simulink model "VCU_SW_2020"  (R2020b)
settings: Solver=FixedStepDiscrete  StartTime=0.0  StopTime=inf  FixedStep=1e-2  RelTol=1e-3
PreLoadFcn:
  | RTWConfigurationCB('preloadfcn', bdroot);
InitFcn:
  | loadvar_ttc500
undefined symbols (not defined in the file): BrkPedalTypes, CabMovModeTypes, cFuseTempSensAcc_X, cFuseTempSensAcc_Y, cFuseTempSensVal_X, cFuseTempSensVal_Y, cTMSTempSensVal_X, cTMSTempSensVal_Y, cTransferCaseSpeedRatio, diag_state, DoorsPositionTypes, dP_filter_Y, DriverOccClassSystemTypes, ErrorValueTypes, fatal_error_callback, IO_ADC_NO_RANGE, LadderStatusTypes, pAnalogCabRotSensAcc, pAnalogCabRotSensMaxVolt, pAnalogCabRotSensMinVolt, pAnalogCabRotSensRange, pAnalogCabRotSensZeroVolt, pBrkActivePress, pCabTiltSensAcc, pCabTiltSensMaxCur, pCabTiltSensMinCur, pDistanceCorrection, pECANManual_BPNEnable, pECANManual_BPNEnabler_Flag, pFilterSensAccRes, pHDirMaxDiffFrq, pHDirSensHighLvl, pHDirSensLowLvl, pMainGearRatio, pMaxFilterSensRes, pMaxFirstPedalSensValue, pMaxFuseTempSensRes, pMaxPressLoss, pMaxPressSensCurrent, pMaxPressValue, pMaxPressValueHydMotAndPump, pMaxPressValueParkDrain, pMaxSecondPedalSensValue, pMaxTempSensVoltage, pMaxTempValue, pMaxTMSTempSensRes, pMinFilterSensRes, pMinFirstPedalSensValue, pMinFuseTempSensRes, pMinPressLoss, pMinPressSensCurrent, pMinPressValue, pMinSecondPedalSensValue, pMinTempSensVoltage, pMinTempValue, pMinTMSTempSensRes, pMotorRingTeethNum, pPedalSensAccuracyPct, pPedalSensAccuracyVolt, pPressLossTreshhold ... (+20)
libraries: TTlibrary x270, canmsglib x127, simulink x88
(part 4 of 17)

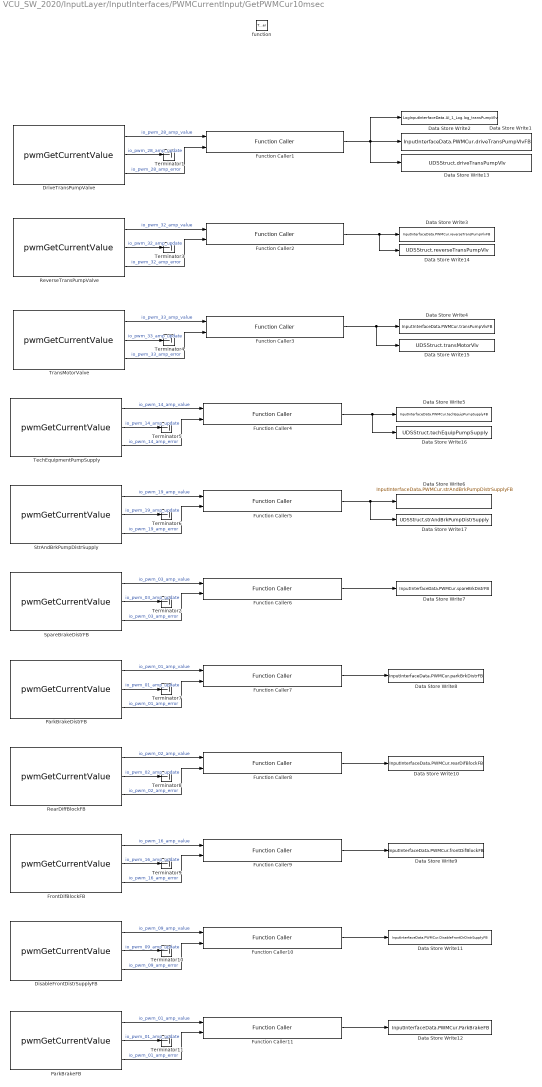
== system VCU_SW_2020/InputLayer/InputInterfaces/PWMCurrentInput/GetPWMCur10msec ==
  function : TriggerPort  TriggerType=function-call  VariantControl=Variant
  Data Store Write1 : DataStoreWrite  DataStoreName=InputInterfaceData  DataStoreElements=InputInterfaceData.PWMCur.driveTransPumpVlvFB
  Data Store Write10 : DataStoreWrite  DataStoreName=InputInterfaceData  DataStoreElements=InputInterfaceData.PWMCur.rearDifBlockFB
  Data Store Write11 : DataStoreWrite  DataStoreName=InputInterfaceData  DataStoreElements=InputInterfaceData.PWMCur.DisableFrontDrDistrSupplyFB
  Data Store Write12 : DataStoreWrite  DataStoreName=InputInterfaceData  DataStoreElements=InputInterfaceData.PWMCur.ParkBrakeFB
  Data Store Write13 : DataStoreWrite  DataStoreName=UDSStruct  DataStoreElements=UDSStruct.driveTransPumpVlv
  Data Store Write14 : DataStoreWrite  DataStoreName=UDSStruct  DataStoreElements=UDSStruct.reverseTransPumpVlv
  Data Store Write15 : DataStoreWrite  DataStoreName=UDSStruct  DataStoreElements=UDSStruct.transMotorVlv
  Data Store Write16 : DataStoreWrite  DataStoreName=UDSStruct  DataStoreElements=UDSStruct.techEquipPumpSupply
  Data Store Write17 : DataStoreWrite  DataStoreName=UDSStruct  DataStoreElements=UDSStruct.strAndBrkPumpDistrSupply
  Data Store Write2 : DataStoreWrite  DataStoreName=LogInputInterfaceData  DataStoreElements=LogInputInterfaceData.AI_1_Log.log_transPumpVlv
  Data Store Write3 : DataStoreWrite  DataStoreName=InputInterfaceData  DataStoreElements=InputInterfaceData.PWMCur.reverseTransPumpVlvFB
  Data Store Write4 : DataStoreWrite  DataStoreName=InputInterfaceData  DataStoreElements=InputInterfaceData.PWMCur.transPumpVlvFB
  Data Store Write5 : DataStoreWrite  DataStoreName=InputInterfaceData  DataStoreElements=InputInterfaceData.PWMCur.techEquipPumpSupplyFB
  Data Store Write6 : DataStoreWrite  DataStoreName=InputInterfaceData  DataStoreElements=InputInterfaceData.PWMCur.strAndBrkPumpDistrSupplyFB
  Data Store Write7 : DataStoreWrite  DataStoreName=InputInterfaceData  DataStoreElements=InputInterfaceData.PWMCur.spareBrkDistrFB
  Data Store Write8 : DataStoreWrite  DataStoreName=InputInterfaceData  DataStoreElements=InputInterfaceData.PWMCur.parkBrkDistrFB
  Data Store Write9 : DataStoreWrite  DataStoreName=InputInterfaceData  DataStoreElements=InputInterfaceData.PWMCur.frontDifBlockFB
  DisableFrontDistrSupplyFB : TTlibrary/PWM /pwmGetCurrentValue  pwm_channel=IO_PWM_09  io_error=on  sample_time=-1
      settings: SourceProductName=TT control 500 series
  DriveTransPumpValve : TTlibrary/PWM /pwmGetCurrentValue  pwm_channel=IO_PWM_28  io_error=on  sample_time=-1
      settings: SourceProductName=TT control 500 series
  FrontDifBlockFB : TTlibrary/PWM /pwmGetCurrentValue  pwm_channel=IO_PWM_16  io_error=on  sample_time=-1
      settings: SourceProductName=TT control 500 series
  Function Caller{1..11} (11 alike) : FunctionCaller  FunctionPrototype=finalValue = convPWMCurrData(rawValue,errorSts)  InputArgumentSpecifications=<Enter example>  OutputArgumentSpecifications=<Enter example>
  ParkBrakeDistrFB : TTlibrary/PWM /pwmGetCurrentValue  pwm_channel=IO_PWM_01  io_error=on  sample_time=-1
      settings: SourceProductName=TT control 500 series
  ParkBrakeFB : TTlibrary/PWM /pwmGetCurrentValue  pwm_channel=IO_PWM_01  io_error=on  sample_time=-1
      settings: SourceProductName=TT control 500 series
  RearDiffBlockFB : TTlibrary/PWM /pwmGetCurrentValue  pwm_channel=IO_PWM_02  io_error=on  sample_time=-1
      settings: SourceProductName=TT control 500 series
  ReverseTransPumpValve : TTlibrary/PWM /pwmGetCurrentValue  pwm_channel=IO_PWM_32  io_error=on  sample_time=-1
      settings: SourceProductName=TT control 500 series
  SpareBrakeDistrFB : TTlibrary/PWM /pwmGetCurrentValue  pwm_channel=IO_PWM_03  io_error=on  sample_time=-1
      settings: SourceProductName=TT control 500 series
  StrAndBrkPumpDistrSupply : TTlibrary/PWM /pwmGetCurrentValue  pwm_channel=IO_PWM_19  io_error=on  sample_time=-1
      settings: SourceProductName=TT control 500 series
  TechEquipmentPumpSupply : TTlibrary/PWM /pwmGetCurrentValue  pwm_channel=IO_PWM_14  io_error=on  sample_time=-1
      settings: SourceProductName=TT control 500 series
  Terminator{1..11} (11 alike) : Terminator
  TransMotorValve : TTlibrary/PWM /pwmGetCurrentValue  pwm_channel=IO_PWM_33  io_error=on  sample_time=-1
      settings: SourceProductName=TT control 500 series
  wires:
  Function Caller7/1 -> Data Store Write8/1
  ParkBrakeDistrFB/2 -> Terminator7/1  "io_pwm_01_amp_update"
  ParkBrakeDistrFB/1 -> Function Caller7/1  "io_pwm_01_amp_value"
  ParkBrakeDistrFB/3 -> Function Caller7/2  "io_pwm_01_amp_error"
  SpareBrakeDistrFB/3 -> Function Caller6/2  "io_pwm_03_amp_error"
  SpareBrakeDistrFB/1 -> Function Caller6/1  "io_pwm_03_amp_value"
  SpareBrakeDistrFB/2 -> Terminator2/1  "io_pwm_03_amp_update"
  Function Caller6/1 -> Data Store Write7/1
  Function Caller1/1 -> Data Store Write13/1, Data Store Write1/1, Data Store Write2/1
  StrAndBrkPumpDistrSupply/3 -> Function Caller5/2  "io_pwm_19_amp_error"
  Function Caller5/1 -> Data Store Write17/1, Data Store Write6/1
  StrAndBrkPumpDistrSupply/1 -> Function Caller5/1  "io_pwm_19_amp_value"
  StrAndBrkPumpDistrSupply/2 -> Terminator6/1  "io_pwm_19_amp_update"
  TechEquipmentPumpSupply/3 -> Function Caller4/2  "io_pwm_14_amp_error"
  Function Caller4/1 -> Data Store Write16/1, Data Store Write5/1
  TechEquipmentPumpSupply/1 -> Function Caller4/1  "io_pwm_14_amp_value"
  TechEquipmentPumpSupply/2 -> Terminator5/1  "io_pwm_14_amp_update"
  TransMotorValve/3 -> Function Caller3/2  "io_pwm_33_amp_error"
  Function Caller3/1 -> Data Store Write15/1, Data Store Write4/1
  TransMotorValve/1 -> Function Caller3/1  "io_pwm_33_amp_value"
  TransMotorValve/2 -> Terminator4/1  "io_pwm_33_amp_update"
  ReverseTransPumpValve/3 -> Function Caller2/2  "io_pwm_32_amp_error"
  Function Caller2/1 -> Data Store Write14/1, Data Store Write3/1
  ReverseTransPumpValve/1 -> Function Caller2/1  "io_pwm_32_amp_value"
  ReverseTransPumpValve/2 -> Terminator3/1  "io_pwm_32_amp_update"
  DriveTransPumpValve/3 -> Function Caller1/2  "io_pwm_28_amp_error"
  DriveTransPumpValve/1 -> Function Caller1/1  "io_pwm_28_amp_value"
  DriveTransPumpValve/2 -> Terminator1/1  "io_pwm_28_amp_update"
  RearDiffBlockFB/2 -> Terminator8/1  "io_pwm_02_amp_update"
  RearDiffBlockFB/3 -> Function Caller8/2  "io_pwm_02_amp_error"
  FrontDifBlockFB/3 -> Function Caller9/2  "io_pwm_16_amp_error"
  FrontDifBlockFB/1 -> Function Caller9/1  "io_pwm_16_amp_value"
  FrontDifBlockFB/2 -> Terminator9/1  "io_pwm_16_amp_update"
  RearDiffBlockFB/1 -> Function Caller8/1  "io_pwm_02_amp_value"
  Function Caller8/1 -> Data Store Write10/1
  Function Caller9/1 -> Data Store Write9/1
  Function Caller10/1 -> Data Store Write11/1
  DisableFrontDistrSupplyFB/2 -> Terminator10/1  "io_pwm_09_amp_update"
  DisableFrontDistrSupplyFB/1 -> Function Caller10/1  "io_pwm_09_amp_value"
  DisableFrontDistrSupplyFB/3 -> Function Caller10/2  "io_pwm_09_amp_error"
  ParkBrakeFB/3 -> Function Caller11/2  "io_pwm_01_amp_error"
  ParkBrakeFB/1 -> Function Caller11/1  "io_pwm_01_amp_value"
  ParkBrakeFB/2 -> Terminator11/1  "io_pwm_01_amp_update"
  Function Caller11/1 -> Data Store Write12/1

== system VCU_SW_2020/InputLayer/InputInterfaces/PWMCurrentInput/PWMCur10msecProc ==
  function : TriggerPort  TriggerType=function-call  VariantControl=Variant
  Constant12 : Constant  Value=pValveActiveCur
  Data Store Read : DataStoreRead  DataStoreName=InputInterfaceData  DataStoreElements=InputInterfaceData.PWMCur.DisableFrontDrDistrSupplyFB
  Data Store Read1 : DataStoreRead  DataStoreName=InputInterfaceData  DataStoreElements=InputInterfaceData.PWMCur.parkBrkDistrFB
  Data Store Read12 : DataStoreRead  DataStoreName=InputInterfaceData  DataStoreElements=InputInterfaceData.PWMCur.spareBrkDistrFB
  Data Store Read2 : DataStoreRead  DataStoreName=InputInterfaceData  DataStoreElements=InputInterfaceData.PWMCur.frontDifBlockFB
  Data Store Read3 : DataStoreRead  DataStoreName=InputInterfaceData  DataStoreElements=InputInterfaceData.PWMCur.rearDifBlockFB
  Data Store Write : DataStoreWrite  DataStoreName=InputFunctionsData  DataStoreElements=InputFunctionsData.frontDifBlockFB
  Data Store Write1 : DataStoreWrite  DataStoreName=InputFunctionsData  DataStoreElements=InputFunctionsData.spareBrkDistrFB
  Data Store Write2 : DataStoreWrite  DataStoreName=InputFunctionsData  DataStoreElements=InputFunctionsData.parkBrkDistrFB
  Data Store Write3 : DataStoreWrite  DataStoreName=InputFunctionsData  DataStoreElements=InputFunctionsData.rearDifBlockFB
  Data Store Write4 : DataStoreWrite  DataStoreName=InputFunctionsData  DataStoreElements=InputFunctionsData.DisableFrontDrDistrSupplyFB
  Data Store Write5 : DataStoreWrite  DataStoreName=InputFunctionsData  DataStoreElements=InputFunctionsData.parkBrakeFB
  Function Caller{,1..4} (5 alike) : FunctionCaller  FunctionPrototype=stt = ValveCurFBproc(pValveActiveCur,curFB)  InputArgumentSpecifications=<Enter example>  OutputArgumentSpecifications=<Enter example>
  MATLAB Function2 : MATLAB Function  TreatAsAtomicUnit=on
  Simulink Function : Subsystem  TreatAsAtomicUnit=on
  wires:
  Constant12/1 -> Function Caller1/1, Function Caller/1, Function Caller2/1, Function Caller3/1, Function Caller4/1
  Function Caller4/1 -> Data Store Write4/1
  Data Store Read/1 -> Function Caller4/2
  Data Store Read3/1 -> Function Caller3/2
  Data Store Read2/1 -> Function Caller2/2
  Function Caller3/1 -> Data Store Write3/1
  Function Caller2/1 -> Data Store Write/1
  Function Caller1/1 -> Data Store Write1/1
  Data Store Read1/1 -> Function Caller/2
  Function Caller/1 -> MATLAB Function2/1(sttRaw), Data Store Write2/1
  Data Store Read12/1 -> Function Caller1/2
  MATLAB Function2/1(sttInv) -> Data Store Write5/1

== system VCU_SW_2020/InputLayer/InputNetwork/InputCCAN/CCAN100msecProc1 ==
  function : TriggerPort  TriggerType=function-call  VariantControl=Variant
  CabMov buttons processing : Subsystem  TreatAsAtomicUnit=on
  InputTransSelect : Subsystem  TreatAsAtomicUnit=on
  JoystickRot : Subsystem  TreatAsAtomicUnit=on

== system VCU_SW_2020/InputLayer/InputNetwork/InputCCAN/CCAN10msecProc  ==
  function : TriggerPort  TriggerType=function-call  VariantControl=Variant

== system VCU_SW_2020/InputLayer/InputNetwork/InputCCAN/GetCCAN1000msec ==
  function : TriggerPort  TriggerType=function-call  VariantControl=Variant
  DD : Subsystem
  "Fuel Heater Data " : Subsystem
  LCMD : Subsystem
  LD : Subsystem
  OCSI : Subsystem
  VF : Subsystem

== system VCU_SW_2020/InputLayer/InputNetwork/InputCCAN/GetCCAN100msec ==
  note: КОСТЫЛЬ
  note: Вот тут тоже с типом данных матлаб функци брехня, посмотреть везде
  function : TriggerPort  TriggerType=function-call  VariantControl=Variant
  AUX_VLV_EST_CABIN : Subsystem
  BJM1 : Subsystem
  BJM2 : Subsystem
  CM1 : Subsystem
  CM3 : Subsystem
  CabinAuxiliaryStatus : Subsystem
  DC1 : Subsystem
  "Fan Rotation Direction Control " : Subsystem
  "Fan Rotation Direction Status " : Subsystem
  FuelTankAndFrameLock : Subsystem
  "Instrument Cluster Status " : Subsystem
  Left Big Pan Cmd : Subsystem
  Left Small Pan Cmd : Subsystem
  "OWW Status " : Subsystem
  PTO : Subsystem
  "Remote Brake Command " : Subsystem
  Right Small Pan Cmd : Subsystem
  TC1 : Subsystem

== system VCU_SW_2020/InputLayer/InputNetwork/InputCCAN/GetCCAN10msec ==
  function : TriggerPort  TriggerType=function-call  VariantControl=Variant
  CAN_Unpack_PLC_StateM : canmsglib/CAN Unpack  Commented=on  MsgList=(none)  MsgName=PLC_StateM  MsgIDType=Extended (29-bit identifier)  MsgIdentifier=419388800  MsgLength=5  SignalInfo={ 'PLC_V2G_StateM_SM9MesState', '16', '8', 'LE', 'unsigned', 'Standard', '0', '1', '0', '0', '255'; 'PLC_V2G_StateM_SM9Status', '24', '8', 'LE', 'unsigned', 'Standard', '0', '1', '0', '0', '255' }  IDPort=off  TimestampPort=off  ErrorPort=off  RemotePort=off  LengthPort=off  StatusPort=off  ApplyMinMax=off
  DataStoreWrite_PLC_StateM : DataStoreWrite  Commented=on  DataStoreName=InputNetworkData  DataStoreElements=InputNetworkData.ECAN.PLC.PLC_V2G_StateM_SM9MesState#InputNetworkData.ECAN.PLC.PLC_V2G_StateM_SM9Status
  Terminator : Terminator  Commented=on
  read_message_PLC_StateM : TTlibrary/CAN/read_message_name  Commented=on  channel=IO_CAN_CHANNEL_1  id_format=IO_CAN_EXT_FRAME  get_msg_info=off  message_names=there is no CAN Unpack blocks  message_info=|  id=419388800  ac_mask=536870911  retranslation=off  io_error=on  sample_time=-1
      | Message Name: PLC_StateM
      |  Message ID Type: Extended (29-bit identifier)
      |  Message ID: 419388800
      settings: SourceProductName=TT control 500 series
  wires:
  read_message_PLC_StateM/1 -> CAN_Unpack_PLC_StateM/1  "msg_419388800"
  read_message_PLC_StateM/2 -> Terminator/1  "handler_err_419388800"
  CAN_Unpack_PLC_StateM/1 -> DataStoreWrite_PLC_StateM/1
  CAN_Unpack_PLC_StateM/2 -> DataStoreWrite_PLC_StateM/2

== system VCU_SW_2020/InputLayer/InputNetwork/InputCCAN/GetCCAN200msec ==
  function : TriggerPort  TriggerType=function-call  VariantControl=Variant
  OWW : Subsystem

== system VCU_SW_2020/InputLayer/InputNetwork/InputCCAN/GetCCAN500msec ==
  function : TriggerPort  TriggerType=function-call  VariantControl=Variant
  EAC1 : Subsystem

== system VCU_SW_2020/InputLayer/InputNetwork/InputDiagCAN/GetDiagCAN10msec ==
  function : TriggerPort  TriggerType=function-call  VariantControl=Variant
  Data Store Write : DataStoreWrite  DataStoreName=UDSStruct  DataStoreElements=UDSStruct.readUDSmsgFlag
  MATLAB Function : MATLAB Function  TreatAsAtomicUnit=on
  Simulink Function : Subsystem  TreatAsAtomicUnit=on
  Simulink Function1 : Subsystem  TreatAsAtomicUnit=on
  Simulink Function2 : Subsystem  TreatAsAtomicUnit=on
  wires:
  MATLAB Function/1(ReadUDSmsgFlag) -> Data Store Write/1

== system VCU_SW_2020/InputLayer/InputNetwork/InputDiagCAN/GetDiagCAN10msec1 ==
  function : TriggerPort  TriggerType=function-call  VariantControl=Variant
  MATLAB Function : MATLAB Function  TreatAsAtomicUnit=on
  Simulink Function1 : Subsystem  TreatAsAtomicUnit=on
  Simulink Function2 : Subsystem  TreatAsAtomicUnit=on

== system VCU_SW_2020/InputLayer/InputNetwork/InputEngCAN/GetEngCAN1000msec ==
  function : TriggerPort  TriggerType=function-call  VariantControl=Variant
  CANUnpack_ECU_DLCC1 : canmsglib/CAN Unpack  MsgList=(none)  MsgName=ECU_DLCC1  MsgIDType=Extended (29-bit identifier)  MsgIdentifier=419235584  MsgLength=8  SignalInfo={ 'ECU_DLCC1_EngAirFiltRestrLampCmd', '22', '2', 'LE', 'unsigned', 'Standard', '0', '1', '0', '0', '3'; 'ECU_DLCC1_EngAmberWarnLampCmd', '2', '2', 'LE', 'unsigned', 'Standard', '0', '1', '0', '0', '3'; 'ECU_DLCC1_EngCoolLevLowLampCmd', '16', '2', 'LE', 'unsigned', 'Standard', '0', '1', '0', '0', '3'; 'ECU_DLCC1_EngCoolTempHiLampCmd', '14', '2', 'LE', 'unsigned', 'Standard', '0', '1', '0', '0', '3'; 'ECU_DLCC1_EngOilPressLowLampCmd', '12', '2', 'LE', 'unsigned', 'Standard', '0', '1', '0', '0', '3'; 'ECU_DLCC1_EngProtLampCmd', '0', '2', 'LE', 'unsigned', 'Standard', '0', '1', '0', '0', '3'; 'ECU_DLCC1_EngRedStopLampCmd', '4', '2', 'LE', 'unsigned', 'Standard', '0', '1', '0', '0', '3' }  IDPort=off  TimestampPort=off  ErrorPort=off  RemotePort=off  LengthPort=off  StatusPort=off  ApplyMinMax=off
  CANUnpack_ECU_ET1 : canmsglib/CAN Unpack  MsgList=(none)  MsgName=ECU_ET1  MsgIDType=Extended (29-bit identifier)  MsgIdentifier=419360256  MsgLength=8  SignalInfo={ 'ECU_ET1_EngCoolTemp', '0', '8', 'LE', 'unsigned', 'Standard', '0', '1', '-40', '-40', '210'; 'ECU_ET1_EngFuelTemp1', '8', '8', 'LE', 'unsigned', 'Standard', '0', '1', '-40', '-40', '210'; 'ECU_ET1_EngIntThOp', '56', '8', 'LE', 'unsigned', 'Standard', '0', '0.4', '0', '0', '100'; 'ECU_ET1_EngInterTemp', '48', '8', 'LE', 'unsigned', 'Standard', '0', '1', '-40', '-40', '210'; 'ECU_ET1_EngOilTemp1', '16', '16', 'LE', 'unsigned', 'Standard', '0', '0.03125', '-273', '-273', '1734.9688'; 'ECU_ET1_EngTurbOilTemp', '32', '16', 'LE', 'unsigned', 'Standard', '0', '0.03125', '-273', '-273', '1734.9688' }  IDPort=off  TimestampPort=off  ErrorPort=off  RemotePort=off  LengthPort=off  StatusPort=off  ApplyMinMax=off
  CANUnpack_ECU_ET2 : canmsglib/CAN Unpack  MsgList=(none)  MsgName=ECU_ET2  MsgIDType=Extended (29-bit identifier)  MsgIdentifier=419341312  MsgLength=8  SignalInfo={ 'ECU_ET2_EngECUTemp', '16', '16', 'LE', 'unsigned', 'Standard', '0', '0.03125', '-273', '-273', '1734.9688'; 'ECU_ET2_EngExGasRec1T', '48', '16', 'LE', 'unsigned', 'Standard', '0', '0.03125', '-273', '-273', '1734.9688'; 'ECU_ET2_EngExhGasRec1DP', '32', '16', 'LE', 'unsigned', 'Standard', '0', '0.0078125', '-250', '-250', '251.99'; 'ECU_ET2_EngOilTemp2', '0', '16', 'LE', 'unsigned', 'Standard', '0', '0.03125', '-273', '-273', '1734.9688' }  IDPort=off  TimestampPort=off  ErrorPort=off  RemotePort=off  LengthPort=off  StatusPort=off  ApplyMinMax=off
  CANUnpack_ECU_ET3 : canmsglib/CAN Unpack  MsgList=(none)  MsgName=ECU_THO  MsgIDType=Extended (29-bit identifier)  MsgIdentifier=419357952  MsgLength=8  SignalInfo={ 'EngTotalHours', '0', '32', 'LE', 'signed', 'Standard', '0', '0.05', '0', '0', '210554060.75' }  IDPort=off  TimestampPort=off  ErrorPort=off  RemotePort=off  LengthPort=off  StatusPort=off  ApplyMinMax=off
  CANUnpack_ECU_SHUTDN : canmsglib/CAN Unpack  MsgList=(none)  MsgName=ECU_SHUTDN  MsgIDType=Extended (29-bit identifier)  MsgIdentifier=419357696  MsgLength=8  SignalInfo={ 'ECU_SHUTDN_ACHighPrFanSw', '16', '2', 'LE', 'unsigned', 'Standard', '0', '1', '0', '0', '3'; 'ECU_SHUTDN_CoolLvlEngPrShSt', '60', '2', 'LE', 'unsigned', 'Standard', '0', '1', '0', '0', '3'; 'ECU_SHUTDN_EnIdShDAM', '2', '2', 'LE', 'unsigned', 'Standard', '0', '1', '0', '0', '3'; 'ECU_SHUTDN_EnIdShSE', '0', '2', 'LE', 'unsigned', 'Standard', '0', '1', '0', '0', '3'; 'ECU_SHUTDN_EnIdShTF', '14', '2', 'LE', 'unsigned', 'Standard', '0', '1', '0', '0', '3'; 'ECU_SHUTDN_EnIdShTO', '4', '2', 'LE', 'unsigned', 'Standard', '0', '1', '0', '0', '3'; 'ECU_SHUTDN_EnIdShTS', '6', '2', 'LE', 'unsigned', 'Standard', '0', '1', '0', '0', '3'; 'ECU_SHUTDN_EngAirShComSt', '52', '2', 'LE', 'unsigned', 'Standard', '0', '1', '0', '0', '3'; 'ECU_SHUTDN_EngAirShSt', '56', '2', 'LE', 'unsigned', 'Standard', '0', '1', '0', '0', '3'; 'ECU_SHUTDN_EngAlAckn', '48', '2', 'LE', 'unsigned', 'Standard', '0', '1', '0', '0', '3'; 'ECU_SHUTDN_EngAlOutComSt', '50', '2', 'LE', 'unsigned', 'Standard', '0', '1', '0', '0', '3'; 'ECU_SHUTDN_EngOverspTest', '54', '2', 'LE', 'unsigned', 'Standard', '0', '1', '0', '0', '3'; 'ECU_SHUTDN_EngProtSysAppSh', '34', '2', 'LE', 'unsigned', 'Standard', '0', '1', '0', '0', '3'; 'ECU_SHUTDN_EngProtSysConf', '46', '2', 'LE', 'unsigned', 'Standard', '0', '1', '0', '0', '3'; 'ECU_SHUTDN_EngProtSysShEng', '32', '2', 'LE', 'unsigned', 'Standard', '0', '1', '0', '0', '3'; 'ECU_SHUTDN_EngProtSysTimOver', '36', '2', 'LE', 'unsigned', 'Standard', '0', '1', '0', '0', '3'; 'ECU_SHUTDN_EngProtSysTimSt', '38', '2', 'LE', 'unsigned', 'Standard', '0', '1', '0', '0', '3'; 'ECU_SHUTDN_EngWaitStLam', '24', '2', 'LE', 'unsigned', 'Standard', '0', '1', '0', '0', '3'; 'ECU_SHUTDN_PTOShSE', '58', '2', 'LE', 'unsigned', 'Standard', '0', '1', '0', '0', '3'; 'ECU_SHUTDN_RefrHiPrSw', '20', '2', 'LE', 'unsigned', 'Standard', '0', '1', '0', '0', '3'; 'ECU_SHUTDN_RefrLowPrSw', '18', '2', 'LE', 'unsigned', 'Standard', '0', '1', '0', '0', '3' }  IDPort=off  TimestampPort=off  ErrorPort=off  RemotePort=off  LengthPort=off  StatusPort=off  ApplyMinMax=off
  CANUnpack_ECU_VEP1 : canmsglib/CAN Unpack  MsgList=(none)  MsgName=ECU_VEP1  MsgIDType=Extended (29-bit identifier)  MsgIdentifier=419362560  MsgLength=8  SignalInfo={ 'ECU_VEP1_AltCur', '8', '8', 'LE', 'unsigned', 'Standard', '0', '1', '-125', '-125', '125'; 'ECU_VEP1_BatPot', '32', '16', 'LE', 'unsigned', 'Standard', '0', '0.05', '0', '0', '3212.75'; 'ECU_VEP1_ChrgSysPot', '16', '16', 'LE', 'unsigned', 'Standard', '0', '0.05', '0', '0', '3212.75'; 'ECU_VEP1_KeyswPot', '48', '16', 'LE', 'unsigned', 'Standard', '0', '0.05', '0', '0', '3212.75'; 'ECU_VEP1_NetBatCur', '0', '8', 'LE', 'unsigned', 'Standard', '0', '1', '-125', '-125', '125' }  IDPort=off  TimestampPort=off  ErrorPort=off  RemotePort=off  LengthPort=off  StatusPort=off  ApplyMinMax=off
  Data Store Write : DataStoreWrite  DataStoreName=InputNetworkData  DataStoreElements=InputNetworkData.EngCAN.EngTotalHours
  Data Store Write1 : DataStoreWrite  DataStoreName=InputNetworkData  DataStoreElements=InputNetworkData.EngCAN.EngAirFiltRestrLampCmd#InputNetworkData.EngCAN.EngAmberWarnLampCmd#InputNetworkData.EngCAN.EngCoolLevLowLampCmd#InputNetworkData.EngCAN.EngCoolTempHiLampCmd#InputNetworkData.EngCAN.EngOilPressLowLampCmd#InputNetworkData.EngCAN.EngProtLampCmd#InputNetworkData.EngCAN.EngRedStopLampCmd
  Data Store Write2 : DataStoreWrite  Commented=on  DataStoreName=InputNetworkData  DataStoreElements=InputNetworkData.EngCAN.EngTotalHours
  Data Store Write4 : DataStoreWrite  DataStoreName=InputNetworkData  DataStoreElements=InputNetworkData.EngCAN.EngCoolTemp#InputNetworkData.EngCAN.EngFuelTemp1#InputNetworkData.EngCAN.EngIntThOp#InputNetworkData.EngCAN.EngInterTemp#InputNetworkData.EngCAN.EngOilTemp1#InputNetworkData.EngCAN.EngTurbOilTemp
  Data Store Write5 : DataStoreWrite  DataStoreName=InputNetworkData  DataStoreElements=InputNetworkData.EngCAN.EngECUTemp#InputNetworkData.EngCAN.EngExGasRec1T#InputNetworkData.EngCAN.EngExhGasRec1DP#InputNetworkData.EngCAN.EngOilTemp2
  Data Store Write6 : DataStoreWrite  DataStoreName=InputNetworkData  DataStoreElements=InputNetworkData.EngCAN.ACHighPrFanSw#InputNetworkData.EngCAN.CoolLvlEngPrShSt#InputNetworkData.EngCAN.EnIdShDAM#InputNetworkData.EngCAN.EnIdShSE#InputNetworkData.EngCAN.EnIdShTF#InputNetworkData.EngCAN.EnIdShTO#InputNetworkData.EngCAN.EnIdShTS#InputNetworkData.EngCAN.EngAirShComSt#InputNetworkData.EngCAN.EngAirShSt#InputNetworkData.EngCAN.EngAlAckn#InputNetworkData.EngCAN.EngAlOutComSt#InputNetworkData.EngCAN.EngOverspTest#InputNetworkData.EngCAN.EngProtSysAppSh#InputNetworkData.EngCAN.EngProtSysConf#InputNetworkData.EngCAN.EngProtSysShEng#InputNetworkData.EngCAN.EngProtSysTimOver#InputNetworkData.EngCAN.EngProtSysTimSt#InputNetworkData.EngCAN.EngWaitStLam#InputNetworkData.EngCAN.PTOShSE#InputNetworkData.EngCAN.RefrHiPrSw#InputNetworkData.EngCAN.RefrLowPrSw
  Data Store Write7 : DataStoreWrite  DataStoreName=InputNetworkData  DataStoreElements=InputNetworkData.EngCAN.AltCur#InputNetworkData.EngCAN.BatPot#InputNetworkData.EngCAN.ChrgSysPot#InputNetworkData.EngCAN.KeyswPot#InputNetworkData.EngCAN.NetBatCur
  Function Caller1 : FunctionCaller  FunctionPrototype=rawValue = convUintPinToenumStt(uintValue)  InputArgumentSpecifications=<Enter example>  OutputArgumentSpecifications=<Enter example>
  MATLAB Function : MATLAB Function  TreatAsAtomicUnit=on
  Terminator{,1..5} (6 alike) : Terminator
  read_DLCC1 : TTlibrary/CAN/read_message_name  channel=IO_CAN_CHANNEL_2  id_format=IO_CAN_EXT_FRAME  get_msg_info=off  message_names=there is no CAN Unpack blocks  message_info=|  id=419235584  ac_mask=536870911  retranslation=off  io_error=on  sample_time=-1
      | Message Name: ECU_VEP1
      |  Message ID Type: Extended (29-bit identifier)
      |  Message ID: 419362560
      settings: SourceProductName=TT control 500 series
  read_DLCC2 : TTlibrary/CAN/read_message_name  channel=IO_CAN_CHANNEL_2  id_format=IO_CAN_EXT_FRAME  get_msg_info=off  message_names=there is no CAN Unpack blocks  message_info=|  id=419357952  ac_mask=536870911  retranslation=off  io_error=on  sample_time=-1
      | Message Name: ECU_VEP1
      |  Message ID Type: Extended (29-bit identifier)
      |  Message ID: 419362560
      settings: SourceProductName=TT control 500 series
  read_ECU_ET1 : TTlibrary/CAN/read_message_name  channel=IO_CAN_CHANNEL_2  id_format=IO_CAN_EXT_FRAME  get_msg_info=off  message_names=there is no CAN Unpack blocks  message_info=|  id=419360256  ac_mask=536870911  retranslation=off  io_error=on  sample_time=-1
      | Message Name: ECU_ET1
      |  Message ID Type: Extended (29-bit identifier)
      |  Message ID: 419360256
      settings: SourceProductName=TT control 500 series
  read_ECU_ET2 : TTlibrary/CAN/read_message_name  channel=IO_CAN_CHANNEL_2  id_format=IO_CAN_EXT_FRAME  get_msg_info=off  message_names=there is no CAN Unpack blocks  message_info=|  id=419341312  ac_mask=536870911  retranslation=off  io_error=on  sample_time=-1
      | Message Name: ECU_ET2
      |  Message ID Type: Extended (29-bit identifier)
      |  Message ID: 419341312
      settings: SourceProductName=TT control 500 series
  read_ECU_SHUTDN : TTlibrary/CAN/read_message_name  channel=IO_CAN_CHANNEL_2  id_format=IO_CAN_EXT_FRAME  get_msg_info=off  message_names=there is no CAN Unpack blocks  message_info=|  id=419357696  ac_mask=536870911  retranslation=off  io_error=on  sample_time=-1
      | Message Name: ECU_SHUTDN
      |  Message ID Type: Extended (29-bit identifier)
      |  Message ID: 419357696
      settings: SourceProductName=TT control 500 series
  read_ECU_VEP1 : TTlibrary/CAN/read_message_name  channel=IO_CAN_CHANNEL_2  id_format=IO_CAN_EXT_FRAME  get_msg_info=off  message_names=there is no CAN Unpack blocks  message_info=|  id=419362560  ac_mask=536870911  retranslation=off  io_error=on  sample_time=-1
      | Message Name: ECU_VEP1
      |  Message ID Type: Extended (29-bit identifier)
      |  Message ID: 419362560
      settings: SourceProductName=TT control 500 series
  wires:
  CANUnpack_ECU_ET3/1 -> Data Store Write/1
  read_DLCC2/2 -> Terminator5/1  "handler_err_419357952"
  read_DLCC2/1 -> CANUnpack_ECU_ET3/1  "msg_419357952"
  CANUnpack_ECU_DLCC1/7 -> Data Store Write1/7
  CANUnpack_ECU_DLCC1/6 -> Data Store Write1/6
  CANUnpack_ECU_DLCC1/5 -> Data Store Write1/5
  CANUnpack_ECU_DLCC1/4 -> Data Store Write1/4
  CANUnpack_ECU_DLCC1/3 -> Data Store Write1/3
  CANUnpack_ECU_DLCC1/2 -> Data Store Write1/2
  CANUnpack_ECU_DLCC1/1 -> Data Store Write1/1
  read_DLCC1/1 -> CANUnpack_ECU_DLCC1/1  "msg_419235584"
  read_DLCC1/2 -> Terminator4/1  "handler_err_419235584"
  MATLAB Function/1(coolLvlState) -> Data Store Write6/2
  CANUnpack_ECU_ET1/5 -> Data Store Write4/5
  Function Caller1/1 -> Data Store Write6/18
  read_ECU_VEP1/2 -> Terminator3/1  "handler_err_419362560"
  read_ECU_SHUTDN/2 -> Terminator2/1  "handler_err_419357696"
  read_ECU_ET2/2 -> Terminator1/1  "handler_err_419341312"
  read_ECU_ET1/2 -> Terminator/1  "handler_err_419360256"
  CANUnpack_ECU_SHUTDN/13 -> Data Store Write6/13
  CANUnpack_ECU_ET1/3 -> Data Store Write4/3
  CANUnpack_ECU_ET2/1 -> Data Store Write5/1
  CANUnpack_ECU_VEP1/2 -> Data Store Write7/2
  CANUnpack_ECU_SHUTDN/1 -> Data Store Write6/1
  CANUnpack_ECU_VEP1/1 -> Data Store Write7/1
  CANUnpack_ECU_ET1/4 -> Data Store Write4/4
  CANUnpack_ECU_SHUTDN/3 -> Data Store Write6/3
  CANUnpack_ECU_VEP1/5 -> Data Store Write7/5
  CANUnpack_ECU_SHUTDN/2 -> MATLAB Function/1(Value)
  CANUnpack_ECU_ET2/2 -> Data Store Write5/2
  CANUnpack_ECU_ET1/2 -> Data Store Write4/2
  CANUnpack_ECU_ET2/3 -> Data Store Write5/3
  CANUnpack_ECU_ET2/4 -> Data Store Write5/4
  CANUnpack_ECU_SHUTDN/5 -> Data Store Write6/5
  CANUnpack_ECU_SHUTDN/6 -> Data Store Write6/6
  CANUnpack_ECU_SHUTDN/8 -> Data Store Write6/8
  CANUnpack_ECU_SHUTDN/16 -> Data Store Write6/16
  CANUnpack_ECU_SHUTDN/9 -> Data Store Write6/9
  CANUnpack_ECU_SHUTDN/11 -> Data Store Write6/11
  CANUnpack_ECU_SHUTDN/10 -> Data Store Write6/10
  CANUnpack_ECU_SHUTDN/14 -> Data Store Write6/14
  CANUnpack_ECU_ET1/6 -> Data Store Write4/6
  CANUnpack_ECU_SHUTDN/15 -> Data Store Write6/15
  CANUnpack_ECU_SHUTDN/18 -> Function Caller1/1
  CANUnpack_ECU_SHUTDN/21 -> Data Store Write6/21
  CANUnpack_ECU_VEP1/3 -> Data Store Write7/3
  CANUnpack_ECU_VEP1/4 -> Data Store Write7/4
  CANUnpack_ECU_ET1/1 -> Data Store Write4/1
  CANUnpack_ECU_SHUTDN/12 -> Data Store Write6/12
  CANUnpack_ECU_SHUTDN/17 -> Data Store Write6/17
  CANUnpack_ECU_SHUTDN/20 -> Data Store Write6/20
  read_ECU_ET1/1 -> CANUnpack_ECU_ET1/1  "msg_419360256"
  read_ECU_SHUTDN/1 -> CANUnpack_ECU_SHUTDN/1  "msg_419357696"
  CANUnpack_ECU_SHUTDN/19 -> Data Store Write6/19
  CANUnpack_ECU_SHUTDN/4 -> Data Store Write6/4
  read_ECU_VEP1/1 -> CANUnpack_ECU_VEP1/1  "msg_419362560"
  CANUnpack_ECU_SHUTDN/7 -> Data Store Write6/7
  read_ECU_ET2/1 -> CANUnpack_ECU_ET2/1  "msg_419341312"

== system VCU_SW_2020/InputLayer/InputNetwork/InputEngCAN/GetEngCAN100msec ==
  function : TriggerPort  TriggerType=function-call  VariantControl=Variant
  CANUnpack_ECU_EEC1 : canmsglib/CAN Unpack  MsgList=(none)  MsgName=ECU_EEC1  MsgIDType=Extended (29-bit identifier)  MsgIdentifier=217056256  MsgLength=8  SignalInfo={ 'ECU_EEC1_ActEngPTrq', '16', '8', 'LE', 'unsigned', 'Standard', '0', '1', '-125', '-125', '125'; 'ECU_EEC1_ActEngPTrqHighRes', '4', '4', 'LE', 'unsigned', 'Standard', '0', '0.125', '0', '0', '0.875'; 'ECU_EEC1_DrDemEngPTrq', '8', '8', 'LE', 'unsigned', 'Standard', '0', '1', '-125', '-125', '125'; 'ECU_EEC1_EnStrtM', '48', '4', 'LE', 'unsigned', 'Standard', '0', '1', '0', '0', '15'; 'ECU_EEC1_EngDemPercTrq', '56', '8', 'LE', 'unsigned', 'Standard', '0', '1', '-125', '-125', '125'; 'ECU_EEC1_EngSpd', '24', '16', 'LE', 'unsigned', 'Standard', '0', '0.125', '0', '0', '8031.875'; 'ECU_EEC1_EngTrqM', '0', '4', 'LE', 'unsigned', 'Standard', '0', '1', '0', '0', '15'; 'ECU_EEC1_SrsAdr', '40', '8', 'LE', 'unsigned', 'Standard', '0', '1', '0', '0', '255' }  IDPort=off  TimestampPort=off  ErrorPort=off  RemotePort=off  LengthPort=off  StatusPort=off  ApplyMinMax=off
  CANUnpack_ECU_LFE1 : canmsglib/CAN Unpack  MsgList=(none)  MsgName=ECU_LFE1  MsgIDType=Extended (29-bit identifier)  MsgIdentifier=419361280  MsgLength=8  SignalInfo={ 'ECU_LFE1_EngAvrFE', '32', '16', 'LE', 'unsigned', 'Standard', '0', '0.0019531', '0', '0', '125.5'; 'ECU_LFE1_EngFuelRate', '0', '16', 'LE', 'unsigned', 'Standard', '0', '0.05', '0', '0', '3212.75'; 'ECU_LFE1_EngInstFE', '16', '16', 'LE', 'unsigned', 'Standard', '0', '0.0019531', '0', '0', '125.5'; 'ECU_LFE1_EngThrVlv1Pos', '48', '8', 'LE', 'unsigned', 'Standard', '0', '0.4', '0', '0', '100'; 'ECU_LFE1_EngThrVlv2Pos', '56', '8', 'LE', 'unsigned', 'Standard', '0', '0.4', '0', '0', '100' }  IDPort=off  TimestampPort=off  ErrorPort=off  RemotePort=off  LengthPort=off  StatusPort=off  ApplyMinMax=off
  CANUnpack_ECU_TPCM : canmsglib/CAN Unpack  Commented=on  MsgList=(none)  MsgName=ECU_TPCM  MsgIDType=Extended (29-bit identifier)  MsgIdentifier=418184960  MsgLength=8  SignalInfo={ 'ECU_TPCM_ContrByte', '0', '8', 'LE', 'unsigned', 'Standard', '0', '1', '0', '0', '255'; 'ECU_TPCM_MaxNumofPak', '32', '8', 'LE', 'unsigned', 'Standard', '0', '1', '0', '2', '255'; 'ECU_TPCM_NextPakNum', '48', '8', 'LE', 'unsigned', 'Standard', '0', '1', '0', '1', '255'; 'ECU_TPCM_NumPakCanSent', '40', '8', 'LE', 'unsigned', 'Standard', '0', '1', '0', '0', '255'; 'ECU_TPCM_SeqNum', '56', '8', 'LE', 'unsigned', 'Standard', '0', '1', '0', '1', '255'; 'ECU_TPCM_TotMesSize', '8', '16', 'LE', 'unsigned', 'Standard', '0', '1', '0', '9', '1785'; 'ECU_TPCM_TotNumofPak', '24', '8', 'LE', 'unsigned', 'Standard', '0', '1', '0', '2', '255' }  IDPort=off  TimestampPort=off  ErrorPort=off  RemotePort=off  LengthPort=off  StatusPort=off  ApplyMinMax=off
  CANUnpack_ECU_TPDT : canmsglib/CAN Unpack  Commented=on  MsgList=(none)  MsgName=ECU_TPDT  MsgIDType=Extended (29-bit identifier)  MsgIdentifier=418119424  MsgLength=8  SignalInfo={ 'ECU_TPDT_EMS_SeqNum', '0', '8', 'LE', 'unsigned', 'Standard', '0', '1', '0', '1', '255'; 'ECU_TPDT_EMS_byte1', '8', '8', 'LE', 'unsigned', 'Standard', '0', '1', '0', '0', '255'; 'ECU_TPDT_EMS_byte2', '16', '8', 'LE', 'unsigned', 'Standard', '0', '1', '0', '0', '255'; 'ECU_TPDT_EMS_byte3', '24', '8', 'LE', 'unsigned', 'Standard', '0', '1', '0', '0', '255'; 'ECU_TPDT_EMS_byte4', '32', '8', 'LE', 'unsigned', 'Standard', '0', '1', '0', '0', '255'; 'ECU_TPDT_EMS_byte5', '40', '8', 'LE', 'unsigned', 'Standard', '0', '1', '0', '0', '7.20575940379279e+16'; 'ECU_TPDT_EMS_byte6', '48', '8', 'LE', 'unsigned', 'Standard', '0', '1', '0', '0', '255'; 'ECU_TPDT_EMS_byte7', '56', '8', 'LE', 'unsigned', 'Standard', '0', '1', '0', '0', '255' }  IDPort=off  TimestampPort=off  ErrorPort=off  RemotePort=off  LengthPort=off  StatusPort=off  ApplyMinMax=off
  Data Store Write4 : DataStoreWrite  DataStoreName=InputNetworkData  DataStoreElements=InputNetworkData.EngCAN.ActEngPTrq#InputNetworkData.EngCAN.ActEngPTrqHighRes#InputNetworkData.EngCAN.DrDemEngPTrq#InputNetworkData.EngCAN.EnStrtM#InputNetworkData.EngCAN.EngDemPercTrq#InputNetworkData.EngCAN.EngSpd#InputNetworkData.EngCAN.EngTrqM#InputNetworkData.EngCAN.SrsAdr
  Data Store Write5 : DataStoreWrite  DataStoreName=InputNetworkData  DataStoreElements=InputNetworkData.EngCAN.EngAvrFE#InputNetworkData.EngCAN.EngFuelRate#InputNetworkData.EngCAN.EngInstFE#InputNetworkData.EngCAN.EngThrVlv1Pos#InputNetworkData.EngCAN.EngThrVlv2Pos
  Data Store Write6 : DataStoreWrite  Commented=on  DataStoreName=InputNetworkData  DataStoreElements=InputNetworkData.EngCAN.ContrByte#InputNetworkData.EngCAN.MaxNumofPak#InputNetworkData.EngCAN.NextPakNum#InputNetworkData.EngCAN.NumPakCanSent#InputNetworkData.EngCAN.SeqNum#InputNetworkData.EngCAN.TotMesSize#InputNetworkData.EngCAN.TotNumofPak
  Data Store Write7 : DataStoreWrite  Commented=on  DataStoreName=InputNetworkData  DataStoreElements=InputNetworkData.EngCAN.EMS_SeqNum#InputNetworkData.EngCAN.EMS_byte1#InputNetworkData.EngCAN.EMS_byte2#InputNetworkData.EngCAN.EMS_byte3#InputNetworkData.EngCAN.EMS_byte4#InputNetworkData.EngCAN.EMS_byte5#InputNetworkData.EngCAN.EMS_byte6#InputNetworkData.EngCAN.EMS_byte7
  Data Type Conversion : DataTypeConversion  OutDataTypeStr=int8
  Data Type Conversion1 : DataTypeConversion  OutDataTypeStr=int8
  Data Type Conversion2 : DataTypeConversion  OutDataTypeStr=int8
  Terminator : Terminator
  Terminator1 : Terminator
  Terminator2 : Terminator  Commented=on
  Terminator3 : Terminator  Commented=on
  calcEnStrtM : MATLAB Function  TreatAsAtomicUnit=on
  read_ECU_EEC1 : TTlibrary/CAN/read_message_name  channel=IO_CAN_CHANNEL_2  id_format=IO_CAN_EXT_FRAME  get_msg_info=off  message_names=there is no CAN Unpack blocks  message_info=|  id=217056256  ac_mask=536870911  retranslation=off  io_error=on  sample_time=-1
      | Message Name: ECU_EEC1
      |  Message ID Type: Extended (29-bit identifier)
      |  Message ID: 217056256
      settings: SourceProductName=TT control 500 series
  read_ECU_LFE1 : TTlibrary/CAN/read_message_name  channel=IO_CAN_CHANNEL_2  id_format=IO_CAN_EXT_FRAME  get_msg_info=off  message_names=there is no CAN Unpack blocks  message_info=|  id=419361280  ac_mask=536870911  retranslation=off  io_error=on  sample_time=-1
      | Message Name: ECU_LFE1
      |  Message ID Type: Extended (29-bit identifier)
      |  Message ID: 419361280
      settings: SourceProductName=TT control 500 series
  read_ECU_TPCM : TTlibrary/CAN/read_message_name  Commented=on  channel=IO_CAN_CHANNEL_2  id_format=IO_CAN_EXT_FRAME  get_msg_info=off  message_names=there is no CAN Unpack blocks  message_info=|  id=418184960  ac_mask=536870911  retranslation=off  io_error=on  sample_time=-1
      | Message Name: ECU_TPCM
      |  Message ID Type: Extended (29-bit identifier)
      |  Message ID: 418184960
      settings: SourceProductName=TT control 500 series
  read_ECU_TPDT : TTlibrary/CAN/read_message_name  Commented=on  channel=IO_CAN_CHANNEL_2  id_format=IO_CAN_EXT_FRAME  get_msg_info=off  message_names=there is no CAN Unpack blocks  message_info=|  id=418119424  ac_mask=536870911  retranslation=off  io_error=on  sample_time=-1
      | Message Name: ECU_TPDT
      |  Message ID Type: Extended (29-bit identifier)
      |  Message ID: 418119424
      settings: SourceProductName=TT control 500 series
  wires:
  CANUnpack_ECU_EEC1/6 -> Data Store Write4/6
  CANUnpack_ECU_EEC1/7 -> Data Store Write4/7
  calcEnStrtM/1(operatingMode) -> Data Store Write4/4
  read_ECU_TPDT/2 -> Terminator3/1  "handler_err_418119424"
  read_ECU_TPCM/2 -> Terminator2/1  "handler_err_418184960"
  read_ECU_LFE1/2 -> Terminator1/1  "handler_err_419361280"
  read_ECU_EEC1/2 -> Terminator/1  "handler_err_217056256"
  CANUnpack_ECU_EEC1/5 -> Data Type Conversion2/1
  CANUnpack_ECU_TPCM/1 -> Data Store Write6/1
  CANUnpack_ECU_EEC1/3 -> Data Type Conversion1/1
  CANUnpack_ECU_TPCM/5 -> Data Store Write6/5
  CANUnpack_ECU_TPDT/3 -> Data Store Write7/3
  CANUnpack_ECU_EEC1/2 -> Data Store Write4/2
  CANUnpack_ECU_TPDT/2 -> Data Store Write7/2
  CANUnpack_ECU_LFE1/2 -> Data Store Write5/2
  CANUnpack_ECU_TPDT/1 -> Data Store Write7/1
  CANUnpack_ECU_TPCM/3 -> Data Store Write6/3
  CANUnpack_ECU_EEC1/4 -> calcEnStrtM/1(Value)
  CANUnpack_ECU_TPDT/6 -> Data Store Write7/6
  CANUnpack_ECU_LFE1/4 -> Data Store Write5/4
  CANUnpack_ECU_TPCM/6 -> Data Store Write6/6
  CANUnpack_ECU_TPCM/2 -> Data Store Write6/2
  CANUnpack_ECU_EEC1/8 -> Data Store Write4/8
  CANUnpack_ECU_TPDT/8 -> Data Store Write7/8
  read_ECU_EEC1/1 -> CANUnpack_ECU_EEC1/1  "msg_217056256"
  CANUnpack_ECU_TPDT/4 -> Data Store Write7/4
  CANUnpack_ECU_TPDT/5 -> Data Store Write7/5
  CANUnpack_ECU_TPCM/4 -> Data Store Write6/4
  CANUnpack_ECU_LFE1/3 -> Data Store Write5/3
  read_ECU_TPCM/1 -> CANUnpack_ECU_TPCM/1  "msg_418184960"
  CANUnpack_ECU_TPDT/7 -> Data Store Write7/7
  CANUnpack_ECU_TPCM/7 -> Data Store Write6/7
  read_ECU_LFE1/1 -> CANUnpack_ECU_LFE1/1  "msg_419361280"
  CANUnpack_ECU_LFE1/5 -> Data Store Write5/5
  CANUnpack_ECU_EEC1/1 -> Data Type Conversion/1
  CANUnpack_ECU_LFE1/1 -> Data Store Write5/1
  read_ECU_TPDT/1 -> CANUnpack_ECU_TPDT/1  "msg_418119424"
  Data Type Conversion/1 -> Data Store Write4/1
  Data Type Conversion1/1 -> Data Store Write4/3
  Data Type Conversion2/1 -> Data Store Write4/5

== system VCU_SW_2020/InputLayer/InputNetwork/InputEngCAN/GetEngCAN250msec ==
  function : TriggerPort  TriggerType=function-call  VariantControl=Variant
  CANUnpack_ECU_EEC3 : canmsglib/CAN Unpack  MsgList=(none)  MsgName=ECU_EEC3  MsgIDType=Extended (29-bit identifier)  MsgIdentifier=419356416  MsgLength=8  SignalInfo={ 'ECU_EEC3_Aft1ExDP', '58', '2', 'LE', 'unsigned', 'Standard', '0', '1', '0', '0', '3'; 'ECU_EEC3_Aft1ExGasMasFl', '40', '16', 'LE', 'unsigned', 'Standard', '0', '0.2', '0', '0', '12851'; 'ECU_EEC3_Aft1IntDP', '56', '2', 'LE', 'unsigned', 'Standard', '0', '1', '0', '0', '3'; 'ECU_EEC3_Aft2ExDP', '62', '2', 'LE', 'unsigned', 'Standard', '0', '1', '0', '0', '3'; 'ECU_EEC3_Aft2IntDP', '60', '2', 'LE', 'unsigned', 'Standard', '0', '1', '0', '0', '3'; 'ECU_EEC3_EngDesOpSpd', '8', '16', 'LE', 'unsigned', 'Standard', '0', '0.125', '0', '0', '8031.875'; 'ECU_EEC3_EngDesOpSpdAA', '24', '8', 'LE', 'unsigned', 'Standard', '0', '1', '0', '0', '250'; 'ECU_EEC3_EstEngParLos', '32', '8', 'LE', 'unsigned', 'Standard', '0', '1', '-125', '-125', '125'; 'ECU_EEC3_NomFrPT', '0', '8', 'LE', 'unsigned', 'Standard', '0', '1', '-125', '-125', '125' }  IDPort=off  TimestampPort=off  ErrorPort=off  RemotePort=off  LengthPort=off  StatusPort=off  ApplyMinMax=off
  Data Store Write4 : DataStoreWrite  DataStoreName=InputNetworkData  DataStoreElements=InputNetworkData.EngCAN.Aft1ExDP#InputNetworkData.EngCAN.Aft1ExGasMasFl#InputNetworkData.EngCAN.Aft1IntDP#InputNetworkData.EngCAN.Aft2ExDP#InputNetworkData.EngCAN.Aft2IntDP#InputNetworkData.EngCAN.EngDesOpSpd#InputNetworkData.EngCAN.EngDesOpSpdAA#InputNetworkData.EngCAN.EstEngParLos#InputNetworkData.EngCAN.NomFrPT
  Terminator : Terminator
  read_ECU_EEC3 : TTlibrary/CAN/read_message_name  channel=IO_CAN_CHANNEL_2  id_format=IO_CAN_EXT_FRAME  get_msg_info=off  message_names=there is no CAN Unpack blocks  message_info=|  id=419356416  ac_mask=536870911  retranslation=off  io_error=on  sample_time=-1
      | Message Name: ECU_EEC3
      |  Message ID Type: Extended (29-bit identifier)
      |  Message ID: 419356416
      settings: SourceProductName=TT control 500 series
  wires:
  read_ECU_EEC3/2 -> Terminator/1  "handler_err_419356416"
  CANUnpack_ECU_EEC3/2 -> Data Store Write4/2
  read_ECU_EEC3/1 -> CANUnpack_ECU_EEC3/1  "msg_419356416"
  CANUnpack_ECU_EEC3/4 -> Data Store Write4/4
  CANUnpack_ECU_EEC3/7 -> Data Store Write4/7
  CANUnpack_ECU_EEC3/1 -> Data Store Write4/1
  CANUnpack_ECU_EEC3/6 -> Data Store Write4/6
  CANUnpack_ECU_EEC3/9 -> Data Store Write4/9
  CANUnpack_ECU_EEC3/8 -> Data Store Write4/8
  CANUnpack_ECU_EEC3/3 -> Data Store Write4/3
  CANUnpack_ECU_EEC3/5 -> Data Store Write4/5

== system VCU_SW_2020/InputLayer/InputNetwork/InputEngCAN/GetEngCAN500msec ==
  function : TriggerPort  TriggerType=function-call  VariantControl=Variant
  CANUnpack_ECU_EFL_P1 : canmsglib/CAN Unpack  MsgList=(none)  MsgName=ECU_EFL_P1  MsgIDType=Extended (29-bit identifier)  MsgIdentifier=419360512  MsgLength=8  SignalInfo={ 'EngCoolLevel', '56', '8', 'LE', 'unsigned', 'Standard', '0', '0.4', '0', '0', '100'; 'EngOilPress', '24', '8', 'LE', 'unsigned', 'Standard', '0', '4', '0', '0', '1000' }  IDPort=off  TimestampPort=off  ErrorPort=off  RemotePort=off  LengthPort=off  StatusPort=off  ApplyMinMax=off
  Data Store Write2 : DataStoreWrite  DataStoreName=InputNetworkData  DataStoreElements=InputNetworkData.EngCAN.EngCoolLevel#InputNetworkData.EngCAN.EngOilPress
  Terminator5 : Terminator
  read_ECU_EFL_P1 : TTlibrary/CAN/read_message_name  channel=IO_CAN_CHANNEL_2  id_format=IO_CAN_EXT_FRAME  get_msg_info=off  message_names=there is no CAN Unpack blocks  message_info=|  id=419360512  ac_mask=536870911  retranslation=off  io_error=on  sample_time=-1
      | Message Name: ECU_VEP1
      |  Message ID Type: Extended (29-bit identifier)
      |  Message ID: 419362560
      settings: SourceProductName=TT control 500 series
  wires:
  CANUnpack_ECU_EFL_P1/2 -> Data Store Write2/2
  CANUnpack_ECU_EFL_P1/1 -> Data Store Write2/1
  read_ECU_EFL_P1/2 -> Terminator5/1  "handler_err_419360512"
  read_ECU_EFL_P1/1 -> CANUnpack_ECU_EFL_P1/1  "msg_419360512"

== system VCU_SW_2020/InputLayer/InputNetwork/InputEngCAN/GetEngCAN50msec ==
  function : TriggerPort  TriggerType=function-call  VariantControl=Variant
  CANUnpack_ECU_EEC2 : canmsglib/CAN Unpack  MsgList=(none)  MsgName=ECU_EEC2  MsgIDType=Extended (29-bit identifier)  MsgIdentifier=217056000  MsgLength=8  SignalInfo={ 'ECU_EEC2_AccPed1LIS', '0', '2', 'LE', 'unsigned', 'Standard', '0', '1', '0', '0', '3'; 'ECU_EEC2_AccPed2LIS', '6', '2', 'LE', 'unsigned', 'Standard', '0', '1', '0', '0', '3'; 'ECU_EEC2_AccPedKS', '2', '2', 'LE', 'unsigned', 'Standard', '0', '1', '0', '0', '3'; 'ECU_EEC2_AccPedPos1', '8', '8', 'LE', 'unsigned', 'Standard', '0', '0.4', '0', '0', '100'; 'ECU_EEC2_AccPedPos2', '32', '8', 'LE', 'unsigned', 'Standard', '0', '0.4', '0', '0', '100'; 'ECU_EEC2_ActMacAvEngTrq', '48', '8', 'LE', 'unsigned', 'Standard', '0', '0.4', '0', '0', '100'; 'ECU_EEC2_DPF', '44', '2', 'LE', 'unsigned', 'Standard', '0', '1', '0', '0', '3'; 'ECU_EEC2_EngPercLoatCS', '16', '8', 'LE', 'unsigned', 'Standard', '0', '1', '0', '0', '250'; 'ECU_EEC2_EstPumpTrq', '56', '8', 'LE', 'unsigned', 'Standard', '0', '1', '-125', '-125', '125'; 'ECU_EEC2_MomEngMaxPwr', '42', '2', 'LE', 'unsigned', 'Standard', '0', '1', '0', '0', '3'; 'ECU_EEC2_RdSpdLS', '4', '2', 'LE', 'unsigned', 'Standard', '0', '1', '0', '0', '3'; 'ECU_EEC2_RemAccPedPos', '24', '8', 'LE', 'unsigned', 'Standard', '0', '0.4', '0', '0', '100'; 'ECU_EEC2_SCR', '46', '2', 'LE', 'unsigned', 'Standard', '0', '1', '0', '0', '3'; 'ECU_EEC2_VehAccRateLimSts', '40', '2', 'LE', 'unsigned', 'Standard', '0', '1', '0', '0', '3' }  IDPort=off  TimestampPort=off  ErrorPort=off  RemotePort=off  LengthPort=off  StatusPort=off  ApplyMinMax=off
  Data Store Write4 : DataStoreWrite  DataStoreName=InputNetworkData  DataStoreElements=InputNetworkData.EngCAN.AccPed1LIS#InputNetworkData.EngCAN.AccPed2LIS#InputNetworkData.EngCAN.AccPedKS#InputNetworkData.EngCAN.AccPedPos1#InputNetworkData.EngCAN.AccPedPos2#InputNetworkData.EngCAN.ActMacAvEngTrq#InputNetworkData.EngCAN.DPF#InputNetworkData.EngCAN.EngPercLoatCS#InputNetworkData.EngCAN.EstPumpTrq#InputNetworkData.EngCAN.MomEngMaxPwr#InputNetworkData.EngCAN.RdSpdLS#InputNetworkData.EngCAN.RemAccPedPos#InputNetworkData.EngCAN.SCR#InputNetworkData.EngCAN.VehAccRateLimSts
  Terminator : Terminator
  read_ECU_EEC2 : TTlibrary/CAN/read_message_name  channel=IO_CAN_CHANNEL_2  id_format=IO_CAN_EXT_FRAME  get_msg_info=off  message_names=there is no CAN Unpack blocks  message_info=|  id=217056000  ac_mask=536870911  retranslation=off  io_error=on  sample_time=-1
      | Message Name: ECU_EEC2
      |  Message ID Type: Extended (29-bit identifier)
      |  Message ID: 217056000
      settings: SourceProductName=TT control 500 series
  wires:
  read_ECU_EEC2/2 -> Terminator/1  "handler_err_217056000"
  CANUnpack_ECU_EEC2/12 -> Data Store Write4/12
  CANUnpack_ECU_EEC2/11 -> Data Store Write4/11
  CANUnpack_ECU_EEC2/13 -> Data Store Write4/13
  CANUnpack_ECU_EEC2/10 -> Data Store Write4/10
  CANUnpack_ECU_EEC2/3 -> Data Store Write4/3
  CANUnpack_ECU_EEC2/8 -> Data Store Write4/8
  CANUnpack_ECU_EEC2/9 -> Data Store Write4/9
  CANUnpack_ECU_EEC2/1 -> Data Store Write4/1
  CANUnpack_ECU_EEC2/4 -> Data Store Write4/4
  CANUnpack_ECU_EEC2/6 -> Data Store Write4/6
  CANUnpack_ECU_EEC2/2 -> Data Store Write4/2
  CANUnpack_ECU_EEC2/14 -> Data Store Write4/14
  CANUnpack_ECU_EEC2/7 -> Data Store Write4/7
  CANUnpack_ECU_EEC2/5 -> Data Store Write4/5
  read_ECU_EEC2/1 -> CANUnpack_ECU_EEC2/1  "msg_217056000"

== system VCU_SW_2020/InputLayer/InputNetwork/InputHydCAN/GetHydCAN100msec ==
  function : TriggerPort  TriggerType=function-call  VariantControl=Variant
  Cabine1stLeftHydCylValve : Subsystem
  Cabine2ndRightHydCylValve : Subsystem
  CabineTurningValve : Subsystem

== system VCU_SW_2020/InputLayer/InputNetwork/InputStrCAN/Function-Call Subsystem ==
  function : TriggerPort  TriggerType=function-call  VariantControl=Variant
  Data Store Read : DataStoreRead  DataStoreName=InputNetworkData  DataStoreElements=InputNetworkData.StrCAN.joystickNeutralPosStt#InputNetworkData.StrCAN.joystickFwdPosStt#InputNetworkData.StrCAN.joystickBckwdPosStt#InputNetworkData.StrCAN.joystickPct
  Data Store Write3 : DataStoreWrite  DataStoreName=InputFunctionsData  DataStoreElements=InputFunctionsData.steerJoyPos
  Data Store Write4 : DataStoreWrite  DataStoreName=InputFunctionsData  DataStoreElements=InputFunctionsData.steerJoyDir
  MATLAB Function1 : MATLAB Function  TreatAsAtomicUnit=on
  wires:
  MATLAB Function1/1(pos) -> Data Store Write3/1
  MATLAB Function1/2(dir) -> Data Store Write4/1
  Data Store Read/1 -> MATLAB Function1/1(neutralPos)
  Data Store Read/2 -> MATLAB Function1/2(fwdPos)
  Data Store Read/3 -> MATLAB Function1/3(bckwdPos)
  Data Store Read/4 -> MATLAB Function1/4(absPos)

== system VCU_SW_2020/InputLayer/InputNetwork/InputStrCAN/GetStrCAN100msec ==
  function : TriggerPort  TriggerType=function-call  VariantControl=Variant
  BJM1 : Subsystem
